simulink model "Sensorless_SVPWM_BLDC"  (R2026a)
settings: Solver=FixedStepDiscrete  FixedStep=1e-6
libraries: simulink x1, slpidlib x1
settings Model: Creator=lagsshin  LastModifiedBy=lagsshin

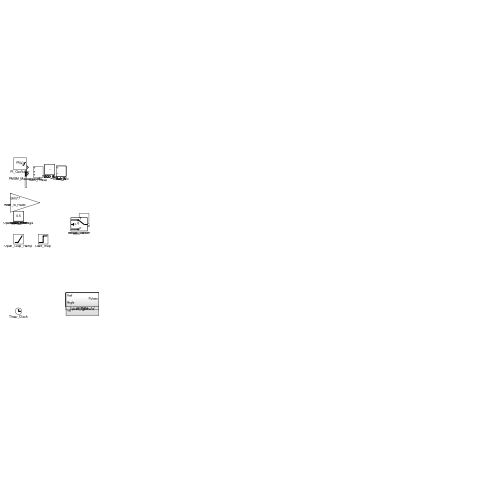
[thumbnail: Simulink's stored preview of the top-level diagram]
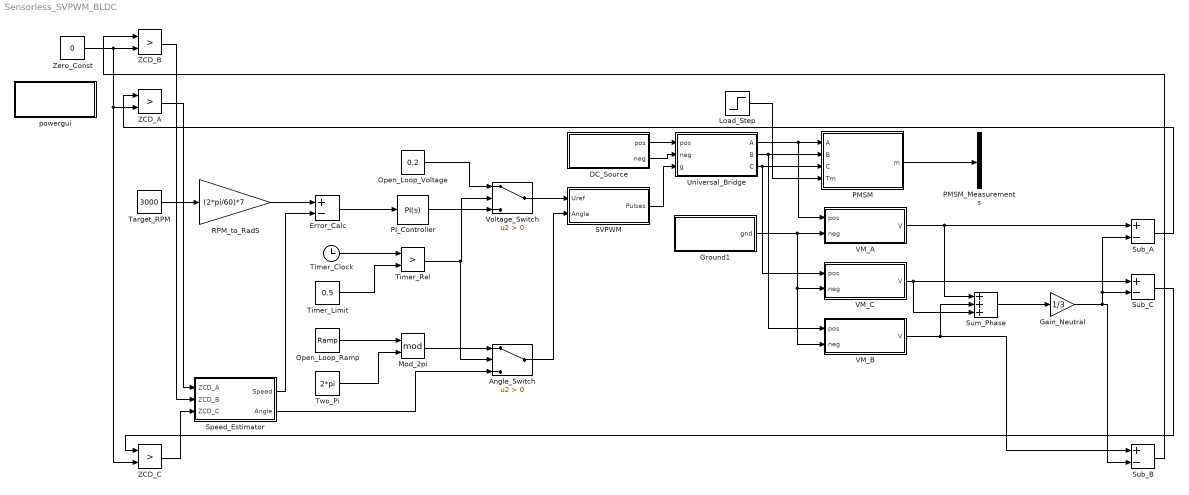
== system Sensorless_SVPWM_BLDC ==
  Angle_Switch : Switch  Criteria=u2 > Threshold  SaturateOnIntegerOverflow=off  InputSameDT=off
  DC_Source : Subsystem
  Error_Calc : Sum  Inputs=+-
  Gain_Neutral : Gain  Gain=1/3
  Ground1 : Subsystem
  Load_Step : Step  Time=1.5  FinalValue=0.05  SampleTime=0
  Mod_2pi : Math  Operator=mod
  Open_Loop_Ramp : simulink/Sources/Ramp  slope=300  start=0  InitialOutput=0
  Open_Loop_Voltage : Constant  Value=0.2
  PI_Controller : slpidlib/PID Controller  Controller=PI  Form=Parallel  TimeDomain=Continuous-time  UseExternalTs=off  SampleTime=-1  IntegratorMethod=Forward Euler  FilterMethod=Forward Euler  ControllerParametersSource=internal  P=1  I=1  UseKiTs=off  D=0  UseExternalDerivativeSource=off  N=100  UseFilter=on  TunerSelectOption=Transfer Function Based (PID Tuner App)  InitialConditionSource=internal  InitialConditionForIntegrator=0  InitialConditionForFilter=0  DifferentiatorICPrevScaledInput=0  ExternalReset=none  TrackingMode=off  Kt=1  LimitOutput=on  SatLimitsSource=internal  UpperSaturationLimit=1.0  LowerSaturationLimit=0.0  LinearizeAsGain=on  AntiWindupMode=none  Kb=1  LimitIntegrator=off  UpperIntegratorSaturationLimit=inf  LowerIntegratorSaturationLimit=-inf  POutMin=[]  POutMax=[]  IOutMin=[]  IOutMax=[]  DOutMin=[]  DOutMax=[]  NOutMin=[]  NOutMax=[]  SumOutMin=[]  SumOutMax=[]  SaturationOutMin=[]  SaturationOutMax=[]  PParamMin=[]  PParamMax=[]  IParamMin=[]  IParamMax=[]  DParamMin=[]  DParamMax=[]  NParamMin=[]  NParamMax=[]  KbParamMin=[]  KbParamMax=[]  KtParamMin=[]  KtParamMax=[]  KbOutMin=[]  KbOutMax=[]  KtOutMin=[]  KtOutMax=[]  IntegratorOutMin=[]  IntegratorOutMax=[]  FilterOutMin=[]  FilterOutMax=[]  SumI1OutMin=[]  SumI1OutMax=[]  SumI2OutMin=[]  SumI2OutMax=[]  SumI3OutMin=[]  SumI3OutMax=[]  SumI4OutMin=[]  SumI4OutMax=[]  SumDOutMin=[]  SumDOutMax=[]  DifferentiatorOutMin=[]  DifferentiatorOutMax=[]  FilterDiffOutCoefMin=[]  FilterDiffOutCoefMax=[]  ReciprocalOutMin=[]  ReciprocalOutMax=[]  SumDenOutMin=[]  SumDenOutMax=[]  SumNumOutMin=[]  SumNumOutMax=[]  DivideOutMin=[]  DivideOutMax=[]  UdiffTsProdOutMin=[]  UdiffTsProdOutMax=[]  NTsProdOutMin=[]  NTsProdOutMax=[]  UintegralTsProdOutMin=[]  UintegralTsProdOutMax=[]  UngainTsProdOutMin=[]  UngainTsProdOutMax=[]  ClampingZeroOutDataTypeStr=Inherit: Inherit via back propagation  ClampingZeroOutMin=[]  ClampingZeroOutMax=[]  FilterDenConstantOutDataTypeStr=Inherit: Inherit via back propagation  FilterDenConstantOutMin=[]  FilterDenConstantOutMax=[]  PCopyOutDataTypeStr=Inherit: Inherit via back propagation  PCopyOutMin=[]  PCopyOutMax=[]  NCopyOutDataTypeStr=Inherit: Inherit via back propagation  NCopyOutMin=[]  NCopyOutMax=[]  IntegratorContinuousStateAttributes=''  IntegratorStateMustResolveToSignalObject=off  IntegratorRTWStateStorageClass=Auto  FilterContinuousStateAttributes=''  FilterStateMustResolveToSignalObject=off  FilterRTWStateStorageClass=Auto  ParallelPVariant=InternalParameters  IdealPVariant=Disabled  IVariant=InternalParameters  DVariant=Disabled  IntegratorVariant=Continuous  SatVariant=Enabled  AWVariant=Passthrough  PCopyVariant=Disabled  TRVariant=Disabled  FdbkBlocksVariant=Forward  IdealPFdbkVariant=Disabled  SatFdbkVariant=Disabled  DerivativeFilterVariant=Disabled  NVariant=Disabled  NCopyVariant=Disabled_SignalSpec  FilterICVariant=Disabled  IntegratorICVariant=InternalICs  ExternalResetVariant=Disabled  TRSumVariant=Passthrough  SumFdbkVariant=Disabled  SumVariant=Sum_PI  TsampFilterVariant=InternalTs  TsampNgainVariant=Passthrough  TsampIntegralVariant=Disabled_SignalSpec  ExternalSaturationOutDataTypeStr=Inherit: Same as second input  DerivativeSourceVariant=Disabled  PreIntVariant=InternalPreInt
  PMSM : Subsystem
  PMSM_Measurements : BusSelector  OutputSignals=signal1,signal2
  RPM_to_RadS : Gain  Gain=(2*pi/60)*7
  SVPWM : Subsystem
  Speed_Estimator : Subsystem
  Sub_A : Sum  Inputs=+-
  Sub_B : Sum  Inputs=+-
  Sub_C : Sum  Inputs=+-
  Sum_Phase : Sum  Inputs=+++
  Target_RPM : Constant  Value=3000
  Timer_Clock : Clock
  Timer_Limit : Constant  Value=0.5
  Timer_Rel : RelationalOperator  Operator=>  OutDataTypeStr=boolean  RndMeth=Simplest  InputSameDT=off
  Two_Pi : Constant  Value=2*pi
  Universal_Bridge : Subsystem
  VM_A : Subsystem
  VM_B : Subsystem
  VM_C : Subsystem
  Voltage_Switch : Switch  Criteria=u2 > Threshold  SaturateOnIntegerOverflow=off  InputSameDT=off
  ZCD_A : RelationalOperator  Operator=>  OutDataTypeStr=boolean  RndMeth=Simplest  InputSameDT=off
  ZCD_B : RelationalOperator  Operator=>  OutDataTypeStr=boolean  RndMeth=Simplest  InputSameDT=off
  ZCD_C : RelationalOperator  Operator=>  OutDataTypeStr=boolean  RndMeth=Simplest  InputSameDT=off
  Zero_Const : Constant  Value=0
  powergui : Subsystem
  wires:
  Sub_C/1 -> ZCD_C/1
  Gain_Neutral/1 -> Sub_C/2, Sub_A/2, Sub_B/2
  VM_B/1(V) -> Sum_Phase/2, Sub_B/1
  VM_A/1(V) -> Sum_Phase/1, Sub_A/1
  Ground1/1(gnd) -> VM_C/2(neg), VM_B/2(neg), VM_A/2(neg)
  Universal_Bridge/3(C) -> VM_C/1(pos), PMSM/3(C)
  VM_C/1(V) -> Sum_Phase/3, Sub_C/1
  Universal_Bridge/2(B) -> VM_B/1(pos), PMSM/2(B)
  Universal_Bridge/1(A) -> VM_A/1(pos), PMSM/1(A)
  RPM_to_RadS/1 -> Error_Calc/1
  Two_Pi/1 -> Mod_2pi/2
  SVPWM/1(Pulses) -> Universal_Bridge/3(g)
  Sub_A/1 -> ZCD_A/1
  PMSM/1(m) -> PMSM_Measurements/1
  DC_Source/2(neg) -> Universal_Bridge/2(neg)
  PI_Controller/1 -> Voltage_Switch/3
  DC_Source/1(pos) -> Universal_Bridge/1(pos)
  Angle_Switch/1 -> SVPWM/2(Angle)
  Sum_Phase/1 -> Gain_Neutral/1
  Load_Step/1 -> PMSM/4(Tm)
  Voltage_Switch/1 -> SVPWM/1(Uref)
  Target_RPM/1 -> RPM_to_RadS/1
  Mod_2pi/1 -> Angle_Switch/1
  Timer_Rel/1 -> Voltage_Switch/2, Angle_Switch/2
  Open_Loop_Voltage/1 -> Voltage_Switch/1
  Open_Loop_Ramp/1 -> Mod_2pi/1
  Timer_Limit/1 -> Timer_Rel/2
  Timer_Clock/1 -> Timer_Rel/1
  Error_Calc/1 -> PI_Controller/1
  Speed_Estimator/2(Angle) -> Angle_Switch/3
  Zero_Const/1 -> ZCD_C/2, ZCD_A/2, ZCD_B/2
  ZCD_B/1 -> Speed_Estimator/2(ZCD_B)
  Sub_B/1 -> ZCD_B/1
  Speed_Estimator/1(Speed) -> Error_Calc/2
  ZCD_C/1 -> Speed_Estimator/3(ZCD_C)
  ZCD_A/1 -> Speed_Estimator/1(ZCD_A)

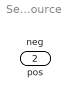
== system Sensorless_SVPWM_BLDC/DC_Source ==
  pos : Outport
  neg : Outport  Port=2

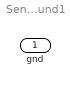
== system Sensorless_SVPWM_BLDC/Ground1 ==
  gnd : Outport

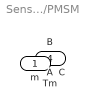
== system Sensorless_SVPWM_BLDC/PMSM ==
  A : Inport
  B : Inport  Port=2
  C : Inport  Port=3
  Tm : Inport  Port=4
  m : Outport

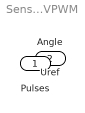
== system Sensorless_SVPWM_BLDC/SVPWM ==
  Uref : Inport
  Angle : Inport  Port=2
  Pulses : Outport

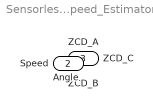
== system Sensorless_SVPWM_BLDC/Speed_Estimator ==
  ZCD_A : Inport
  ZCD_B : Inport  Port=2
  ZCD_C : Inport  Port=3
  Speed : Outport
  Angle : Outport  Port=2

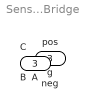
== system Sensorless_SVPWM_BLDC/Universal_Bridge ==
  pos : Inport
  neg : Inport  Port=2
  g : Inport  Port=3
  A : Outport
  B : Outport  Port=2
  C : Outport  Port=3

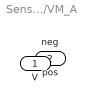
== system Sensorless_SVPWM_BLDC/VM_A ==
  pos : Inport
  neg : Inport  Port=2
  V : Outport

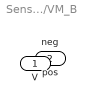
== system Sensorless_SVPWM_BLDC/VM_B ==
  pos : Inport
  neg : Inport  Port=2
  V : Outport

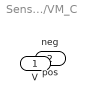
== system Sensorless_SVPWM_BLDC/VM_C ==
  pos : Inport
  neg : Inport  Port=2
  V : Outport

== system Sensorless_SVPWM_BLDC/powergui ==
